simulink model "Lab8_audio_system_toolbox_template"  (R2023b)
settings: Solver=FixedStepDiscrete  StartTime=0.0  StopTime=inf  RelTol=1e-3  EnableMultiTasking=on
libraries: dspfdesign x5, dspsrcs4 x2, audiosources x1, dspsnks4 x1
settings Model: Creator=Student  LastModifiedBy=shaanyadav
settings SolverCC: AlgebraicLoopSolver=TrustRegion  PositivePriorityOrder=on
settings DataIOCC: LimitDataPoints=on  SaveFormat=Array  SaveOutput=off  SaveTime=off  ReturnWorkspaceOutputs=off
settings OptimizationCC: LifeSpan=1
settings DebuggingCC: UnconnectedInputMsg=warning  UnconnectedOutputMsg=warning  UnconnectedLineMsg=warning  SFUnexpectedBacktrackingDiag=warning  SFNoUnconditionalDefaultTransitionDiag=warning  ArithmeticOperatorsInVariantConditions=warning
settings HardwareCC: ProdBitPerLong=40  ProdBitPerPointer=32  ProdBitPerSizeT=32  ProdBitPerPtrDiffT=32  ProdLargestAtomicInteger=Integer  ProdLargestAtomicFloat=None  ProdWordSize=32  ProdHWDeviceType=Texas Instruments->C6000
settings ModelReferenceCC: EnableRefExpFcnMdlSchedulingChecks=on  PropagateSignalLabelsOutOfModel=off
settings SFSimCC: SimUseLocalCustomCode=off  CustomCodeUndefinedFunction=UseInterfaceOnly
settings RTWCC: Description=IDE Link ERT  SystemTargetFile=idelink_ert.tlc  GenerateMakefile=off  TemplateMakefile=none  RTWUseLocalCustomCode=off
settings CodeAppCC: StateflowObjectComments=on
settings TargetCC: CompOptLevelCompliant=off  ConcurrentExecutionCompliant=on  CombineOutputUpdateFcns=on  RemoveResetFunc=on  MATLABClassNameForMDSCustomization=linkfoundation.pjtgenerator.IdelinkCustomization  GRTInterface=off  OptimizeReductions=off
settings ConfigComp: CovMetricSettings=dw  CovSaveCumulativeToWorkspaceVar=on  CovSaveSingleToWorkspaceVar=on  CovExternalEMLEnable=off
settings TargetHardwareResources: Description=Target Hardware Resources Component

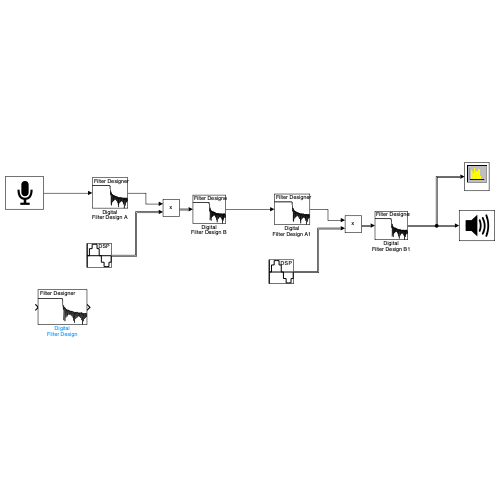
[thumbnail: Simulink's stored preview of the top-level diagram]
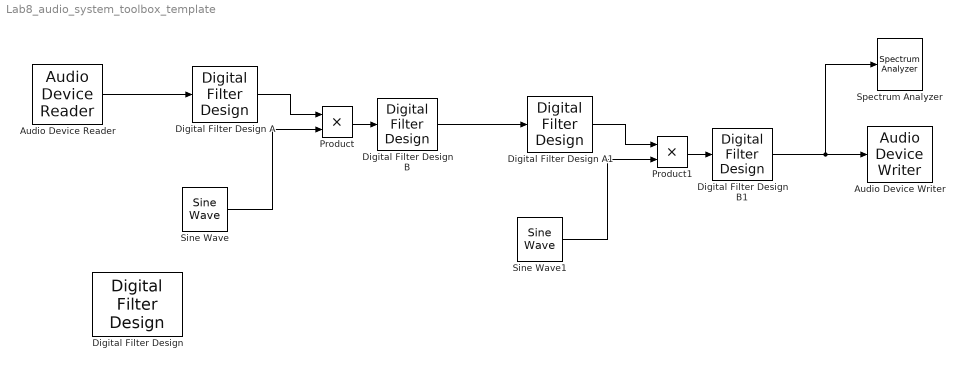
== system Lab8_audio_system_toolbox_template ==
  Audio Device Reader : audiosources/Audio Device Reader  Driver=CoreAudio  Device=Default  SampleRate=8000  NumChannels=1  SamplesPerFrame=1024  BitDepth=16-bit integer  NumBuffers=10  DefaultInputChannelMapping=on  InputChannelMapping=1:2  OutputNumOverrunSamples=off  OutputDataType=double  DriverIdx=5  DeviceWarnFlag=''
  Audio Device Writer : dspsnks4/Audio Device Writer  Driver=CoreAudio  Device=Default  InheritSampleRate=on  SampleRate=44100  BitDepth=16-bit integer  BufferSize=4096  NumBuffers=10  DefaultOutputChannelMapping=on  OutputChannelMapping=1:2  OutputNumUnderrunSamples=off  DriverIdx=5  DeviceWarnFlag=''
  Digital Filter Design : dspfdesign/Digital Filter Design  mwdsp_browser_bugfix_var=off
  Digital Filter Design A : dspfdesign/Digital Filter Design  mwdsp_browser_bugfix_var=off
  Digital Filter Design A1 : dspfdesign/Digital Filter Design  mwdsp_browser_bugfix_var=off
  Digital Filter Design B : dspfdesign/Digital Filter Design  mwdsp_browser_bugfix_var=off
  Digital Filter Design B1 : dspfdesign/Digital Filter Design  mwdsp_browser_bugfix_var=off
  Product : Product  RndMeth=Zero
  Product1 : Product  RndMeth=Zero
  Sine Wave : dspsrcs4/Sine Wave  Amplitude=1  Frequency=2000  Phase=0  SampleMode=Discrete  OutComplex=Real  CompMethod=Trigonometric fcn  TableSize=Speed  SampleTime=1/8000  SamplesPerFrame=1024  ResetState=Restart at time zero  OutputFrames=on  dataType=double  wordLen=16  udDataType=sfix(16)  fracBitsMode=Best precision  numFracBits=15  OutDataTypeStr=double  LastOutDataTypeStr=double
  Sine Wave1 : dspsrcs4/Sine Wave  Amplitude=1  Frequency=2000  Phase=0  SampleMode=Discrete  OutComplex=Real  CompMethod=Trigonometric fcn  TableSize=Speed  SampleTime=1/8000  SamplesPerFrame=1024  ResetState=Restart at time zero  OutputFrames=on  dataType=double  wordLen=16  udDataType=sfix(16)  fracBitsMode=Best precision  numFracBits=15  OutDataTypeStr=double  LastOutDataTypeStr=double
  Spectrum Analyzer : SpectrumAnalyzer  WindowPosition=[276.000000,189.000000,800.000000,500.000000,]  ScopeFrameLocation=window  Method=Welch  SampleRate=8000  Span=8000  StartFrequency=-4000  StopFrequency=4000  AveragingMethod=Running  YLabel=dBm  YLimits=[-161.37538666,-1.56790062]  ShowGrid=off  SelectedToolstripTab=spectrumAnalyzerToolstrip.measurementsTab  DefaultConfigurationName=spbscopes.SpectrumAnalyzerBlockCfg
  wires:
  Audio Device Reader/1 -> Digital Filter Design A/1
  Sine Wave/1 -> Product/2
  Digital Filter Design A/1 -> Product/1
  Product/1 -> Digital Filter Design B/1
  Digital Filter Design B1/1 -> Audio Device Writer/1, Spectrum Analyzer/1
  Sine Wave1/1 -> Product1/2
  Digital Filter Design B/1 -> Digital Filter Design A1/1
  Digital Filter Design A1/1 -> Product1/1
  Product1/1 -> Digital Filter Design B1/1
